simulink model "ctrl_dina_vel_lineal"  (Simulink 9.2)
settings: Solver=ode4  StartTime=0.0  StopTime=30.0  FixedStep=0.05  RelTol=1e-3
settings Model: Creator=hathaway  LastModifiedBy=hathaway
settings DataIOCC: LimitDataPoints=off  SaveFormat=Dataset  SignalLoggingSaveFormat=Dataset
settings OptimizationCC: LifeSpan=auto
settings DebuggingCC: UnderspecifiedInitializationDetection=Simplified  MergeDetectMultiDrivingBlocksExec=error  FcnCallInpInsideContextMsg=error  StateNameClashWarn=none  SFUnexpectedBacktrackingDiag=error  SFNoUnconditionalDefaultTransitionDiag=error  SFExecutionAtInitializationDiag=warning
settings HardwareCC: ProdBitPerPointer=64  ProdBitPerSizeT=64  ProdBitPerPtrDiffT=64  ProdLargestAtomicFloat=Float  ProdIntDivRoundTo=Zero  ProdEndianess=LittleEndian  ProdWordSize=64  ProdHWDeviceType=Intel->x86-64 (Windows64)
settings ModelReferenceCC: PropagateSignalLabelsOutOfModel=on
settings SFSimCC: SimUseLocalCustomCode=on
settings RTWCC: RTWUseLocalCustomCode=on
settings CodeAppCC: StateflowObjectComments=off
settings GRTTargetCC: TargetLangStandard=C99 (ISO)  GeneratePreprocessorConditionals=Use local settings  CombineOutputUpdateFcns=on  GRTInterface=off
settings ConfigComp: CovMetricSettings=dwe  CovHtmlReporting=off  CovSaveCumulativeToWorkspaceVar=off  CovSaveSingleToWorkspaceVar=off  CovExternalEMLEnable=on

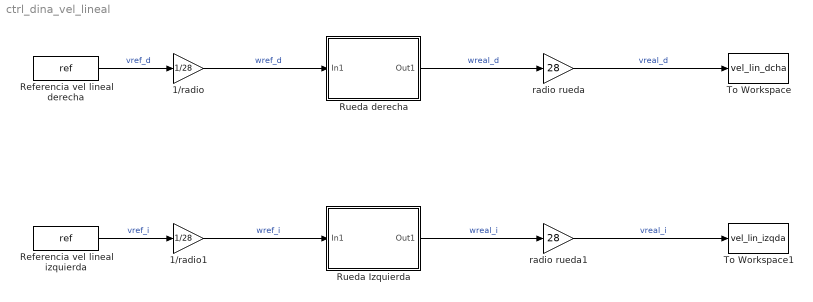
== system ctrl_dina_vel_lineal ==
  1/radio : Gain  Gain=1/28
  1/radio1 : Gain  Gain=1/28
  Referencia vel lineal derecha : FromWorkspace  VariableName=ref  SampleTime=0
  Referencia vel lineal izquierda : FromWorkspace  VariableName=ref  SampleTime=0
  Rueda Izquierda : Subsystem  mask{k=0, tau=0, kp=0}
      mask prompts: k "Valor ganancia del motor:"; tau "Valor cte tiempo motor:"; kp "Valor ganancia regulador P:"
  Rueda derecha : Subsystem  mask{k=0, tau=0, kp=0}
      mask prompts: k "Valor ganancia del motor:"; tau "Valor cte tiempo motor:"; kp "Valor ganancia regulador P:"
  To Workspace : ToWorkspace  VariableName=vel_lin_dcha  SaveFormat=Timeseries  SampleTime=-1
  To Workspace1 : ToWorkspace  VariableName=vel_lin_izqda  SaveFormat=Timeseries  SampleTime=-1
  radio rueda : Gain  Gain=28
  radio rueda1 : Gain  Gain=28
  wires:
  Referencia vel lineal derecha/1 -> 1/radio/1  "vref_d"
  Rueda derecha/1(Out1) -> radio rueda/1  "wreal_d"
  Rueda Izquierda/1(Out1) -> radio rueda1/1  "wreal_i"
  Referencia vel lineal izquierda/1 -> 1/radio1/1  "vref_i"
  1/radio/1 -> Rueda derecha/1(In1)  "wref_d"
  1/radio1/1 -> Rueda Izquierda/1(In1)  "wref_i"
  radio rueda/1 -> To Workspace/1  "vreal_d"
  radio rueda1/1 -> To Workspace1/1  "vreal_i"

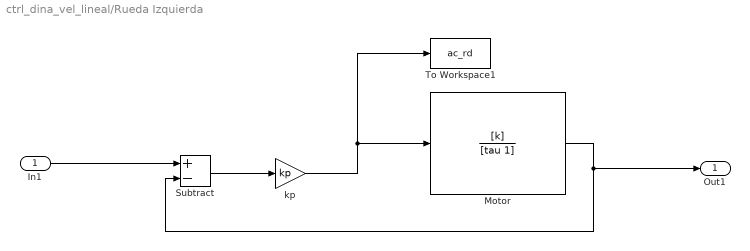
== system ctrl_dina_vel_lineal/Rueda Izquierda ==
  In1 : Inport
  Motor : TransferFcn  Numerator=[k]  Denominator=[tau 1]
  Subtract : Sum  Inputs=+-
  To Workspace1 : ToWorkspace  VariableName=ac_rd  SaveFormat=Timeseries  SampleTime=-1
  kp : Gain  Gain=kp
  Out1 : Outport
  wires:
  In1/1 -> Subtract/1
  Subtract/1 -> kp/1
  kp/1 -> Motor/1, To Workspace1/1
  Motor/1 -> Subtract/2, Out1/1

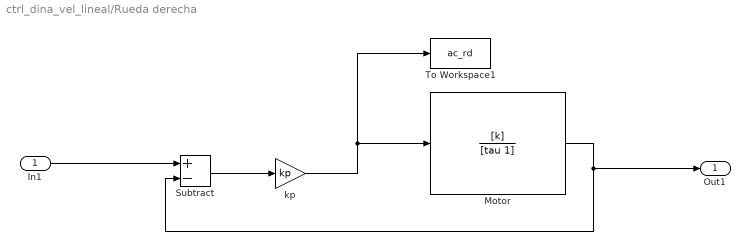
== system ctrl_dina_vel_lineal/Rueda derecha ==
  In1 : Inport
  Motor : TransferFcn  Numerator=[k]  Denominator=[tau 1]
  Subtract : Sum  Inputs=+-
  To Workspace1 : ToWorkspace  VariableName=ac_rd  SaveFormat=Timeseries  SampleTime=-1
  kp : Gain  Gain=kp
  Out1 : Outport
  wires:
  Motor/1 -> Out1/1, Subtract/2
  kp/1 -> To Workspace1/1, Motor/1
  Subtract/1 -> kp/1
  In1/1 -> Subtract/1
